simulink model "test_aero_model"  (R2021b)
settings: Solver=VariableStepAuto  StartTime=0.0  StopTime=20.0  RelTol=1e-3
values from neighbouring files (symbols this model uses):
  A = [0 1; -m*l*g*d/J -c/J]    [custom_env_test.m]
  B = [0; Km/J]    [custom_env_test.m]
  C = [1 0]    [custom_env_test.m]
  yref = 60    [custom_env_test.m]
libraries: rllib x1
settings Model: Creator=Marcin  LastModifiedBy=Marcin

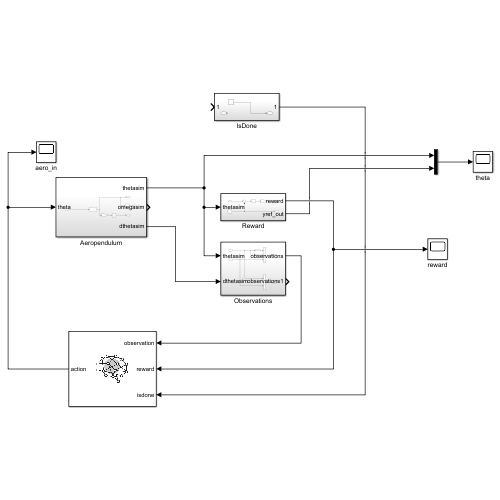
[thumbnail: Simulink's stored preview of the top-level diagram]
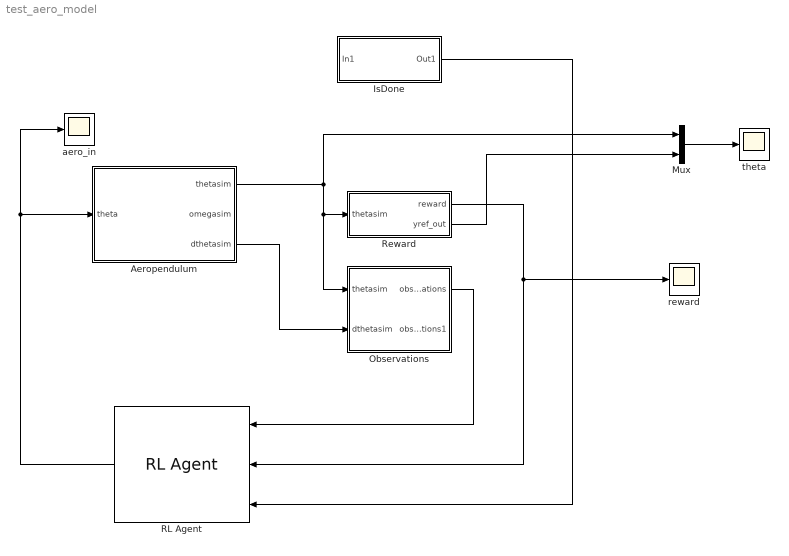
== system test_aero_model ==
  Aeropendulum : Subsystem
  IsDone : Subsystem
  Mux : Mux  Inputs=2
  Observations : Subsystem
  RL Agent : rllib/RL Agent  Agent=agent_aero_v1_Trained  ExternalActionAsInput=off  ProvideCumRwd=off  TreatAsDirectFeedthrough=on
  Reward : Subsystem
  aero_in : Scope
  reward : Scope
  theta : Scope
  wires:
  Observations/1(observations) -> RL Agent/1
  IsDone/1(Out1) -> RL Agent/3
  Reward/1(reward) -> reward/1, RL Agent/2
  Aeropendulum/3(dthetasim) -> Observations/2(dthetasim)
  Aeropendulum/1(thetasim) -> Mux/1, Reward/1(thetasim), Observations/1(thetasim)
  RL Agent/1 -> aero_in/1, Aeropendulum/1(theta)
  Mux/1 -> theta/1
  Reward/2(yref_out) -> Mux/2

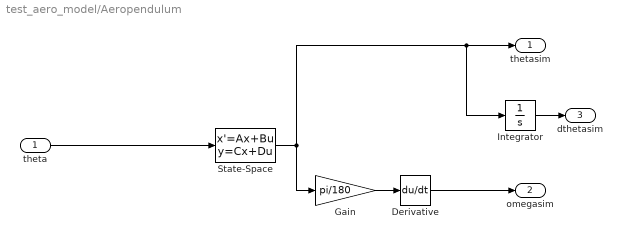
== system test_aero_model/Aeropendulum ==
  theta : Inport
  Derivative : Derivative
  Gain : Gain  Gain=pi/180
  Integrator : Integrator
  State-Space : StateSpace  A=A  B=B  C=C  D=0  InitialCondition=0
  thetasim : Outport
  omegasim : Outport  Port=2
  dthetasim : Outport  Port=3
  wires:
  State-Space/1 -> Integrator/1, thetasim/1, Gain/1
  Gain/1 -> Derivative/1
  theta/1 -> State-Space/1
  Derivative/1 -> omegasim/1
  Integrator/1 -> dthetasim/1

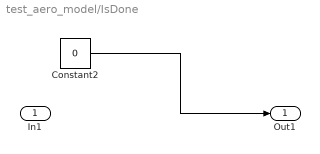
== system test_aero_model/IsDone ==
  In1 : Inport
  Constant2 : Constant  Value=0
  Out1 : Outport
  wires:
  Constant2/1 -> Out1/1

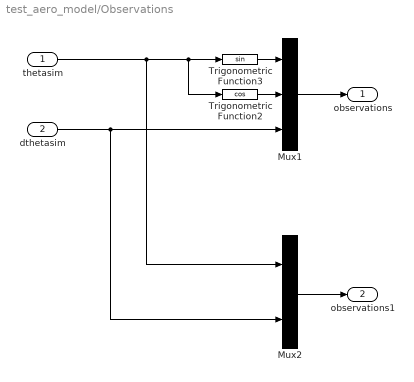
== system test_aero_model/Observations ==
  thetasim : Inport
  dthetasim : Inport  Port=2
  Mux1 : Mux  Inputs=3
  Mux2 : Mux  Inputs=2
  Trigonometric Function2 : Trigonometry  Operator=cos
  Trigonometric Function3 : Trigonometry
  observations : Outport
  observations1 : Outport  Port=2
  wires:
  Trigonometric Function3/1 -> Mux1/1
  dthetasim/1 -> Mux2/2, Mux1/3
  thetasim/1 -> Mux2/1, Trigonometric Function2/1, Trigonometric Function3/1
  Trigonometric Function2/1 -> Mux1/2
  Mux1/1 -> observations/1
  Mux2/1 -> observations1/1

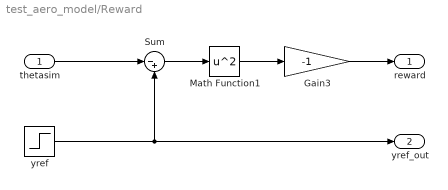
== system test_aero_model/Reward ==
  thetasim : Inport
  Gain3 : Gain  Gain=-1
  Math Function1 : Math  Operator=square  SignedPower=on  SaturateOnIntegerOverflow=on
  Sum : Sum  Inputs=|-+
  yref : Step  Time=0  After=yref  SampleTime=0
  reward : Outport
  yref_out : Outport  Port=2
  wires:
  yref/1 -> yref_out/1, Sum/2
  thetasim/1 -> Sum/1
  Sum/1 -> Math Function1/1
  Math Function1/1 -> Gain3/1
  Gain3/1 -> reward/1
